simulink model "closedloop2017"  (R2017b)
settings: Solver=FixedStepAuto  StartTime=0.0  StopTime=inf  RelTol=1e-3
libraries: arduinolib x3, simulink x1
settings Model: ExtModeTrigDuration=2  Creator=colpari  LastModifiedBy=colpari
settings DataIOCC: ReturnWorkspaceOutputs=on
settings OptimizationCC: EnhancedBackFolding=on  PassReuseOutputArgsAs=Individual arguments  ZeroExternalMemoryAtStartup=off  ZeroInternalMemoryAtStartup=off  MaxStackSize=64  OptimizeBlockOrder=speed  DifferentSizesBufferReuse=on
settings DebuggingCC: ParameterTunabilityLossMsg=error
settings HardwareCC: ProdBitPerInt=16  ProdBitPerPointer=16  ProdBitPerSizeT=16  ProdBitPerPtrDiffT=16  ProdLargestAtomicFloat=None  ProdWordSize=8  ProdHWDeviceType=Atmel->AVR  UseEmbeddedCoderFeatures=off
settings SFSimCC: SimUseLocalCustomCode=on  MATLABDynamicMemAlloc=off
settings RTWCC: SystemTargetFile=ert.tlc  HardwareBoard=Arduino Uno  TLCOptions=-aInlineSetEventsForThisBaseRateFcn=TLC_FALSE -aSuppressMultiTaskScheduler=TLC_FALSE -aRateBasedStepFcn=1  TemplateMakefile=ert_default_tmf  RTWUseLocalCustomCode=on  Toolchain=Arduino AVR
settings CodeAppCC: ForceParamTrailComments=on  IgnoreCustomStorageClasses=off  OperatorAnnotations=on  SimulinkDataObjDesc=on  SFDataObjDesc=on  InsertBlockDesc=on
settings ERTTargetCC: SupportContinuousTime=on  SupportNonInlinedSFcns=on  SupportVariableSizeSignals=on  ExtModeStaticAllocSize=250

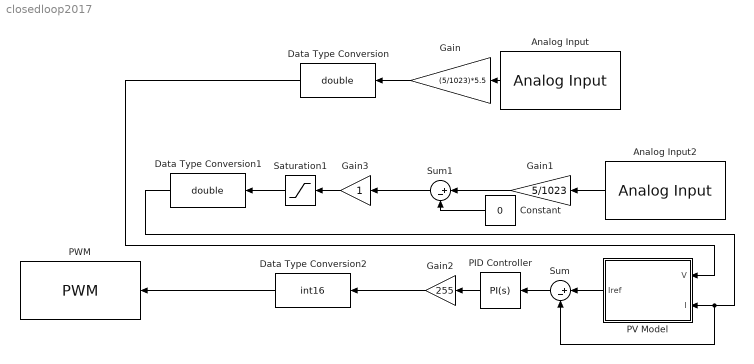
== system closedloop2017 ==
  Analog Input : arduinolib/Analog Input  pinNumber=4  ReadResultsOnly=off  ConversionTriggerSource=Software  ExternalTriggerType=uint32( 0 )  OutputDataType=uint16  EnableConversionCompleteNotify=off  EnableOuputStatus=off  SampleTime=-1  blockPlatform=arduino
  Analog Input2 : arduinolib/Analog Input  pinNumber=5  ReadResultsOnly=off  ConversionTriggerSource=Software  ExternalTriggerType=uint32( 0 )  OutputDataType=uint16  EnableConversionCompleteNotify=off  EnableOuputStatus=off  SampleTime=-1  blockPlatform=arduino
  Constant : Constant  Value=0
  Data Type Conversion : DataTypeConversion  OutDataTypeStr=double
  Data Type Conversion1 : DataTypeConversion  OutDataTypeStr=double
  Data Type Conversion2 : DataTypeConversion  OutDataTypeStr=int16
  Gain : Gain  Gain=(5/1023)*5.5
  Gain1 : Gain  Gain=5/1023
  Gain2 : Gain  Gain=255
  Gain3 : Gain
  PID Controller : simulink/Continuous/PID Controller  Controller=PI  Form=Parallel  TimeDomain=Continuous-time  SampleTime=-1  IntegratorMethod=Forward Euler  FilterMethod=Forward Euler  ControllerParametersSource=internal  P=7  I=0.003  D=0  UseFilter=on  N=100  TunerSelectOption=Transfer Function Based (PID Tuner App)  InitialConditionSource=internal  InitialConditionForIntegrator=0  InitialConditionForFilter=0  DifferentiatorICPrevScaledInput=0  ExternalReset=none  TrackingMode=off  Kt=1  LimitOutput=on  UpperSaturationLimit=1  LowerSaturationLimit=0  LinearizeAsGain=on  AntiWindupMode=none  Kb=1  POutMin=[]  POutMax=[]  IOutMin=[]  IOutMax=[]  DOutMin=[]  DOutMax=[]  NOutMin=[]  NOutMax=[]  SumOutMin=[]  SumOutMax=[]  SaturationOutMin=[]  SaturationOutMax=[]  PParamMin=[]  PParamMax=[]  IParamMin=[]  IParamMax=[]  DParamMin=[]  DParamMax=[]  NParamMin=[]  NParamMax=[]  KbParamMin=[]  KbParamMax=[]  KtParamMin=[]  KtParamMax=[]  KbOutMin=[]  KbOutMax=[]  KtOutMin=[]  KtOutMax=[]  IntegratorOutMin=[]  IntegratorOutMax=[]  FilterOutMin=[]  FilterOutMax=[]  SumI1OutMin=[]  SumI1OutMax=[]  SumI2OutMin=[]  SumI2OutMax=[]  SumI3OutMin=[]  SumI3OutMax=[]  SumDOutMin=[]  SumDOutMax=[]  DifferentiatorOutMin=[]  DifferentiatorOutMax=[]  FilterDiffOutCoefMin=[]  FilterDiffOutCoefMax=[]  ReciprocalOutMin=[]  ReciprocalOutMax=[]  SumDenOutMin=[]  SumDenOutMax=[]  SumNumOutMin=[]  SumNumOutMax=[]  DivideOutMin=[]  DivideOutMax=[]  IntegratorContinuousStateAttributes=''  IntegratorStateMustResolveToSignalObject=off  IntegratorRTWStateStorageClass=Auto  FilterContinuousStateAttributes=''  FilterStateMustResolveToSignalObject=off  FilterRTWStateStorageClass=Auto  InitialConditionSetting=State (most efficient)
  PV Model : Subsystem
  PWM : arduinolib/PWM  pinNumber=11  frequencyType=Specify  desiredFrequency=3921.16  achievableFrequency=3921.16
  Saturation1 : Saturate  LowerLimit=0
  Sum : Sum  Inputs=|+-
  Sum1 : Sum  Inputs=|+-
  wires:
  Analog Input/1 -> Gain/1
  Analog Input2/1 -> Gain1/1
  Gain/1 -> Data Type Conversion/1
  Saturation1/1 -> Data Type Conversion1/1
  Data Type Conversion2/1 -> PWM/1
  Gain2/1 -> Data Type Conversion2/1
  PID Controller/1 -> Gain2/1
  Data Type Conversion/1 -> PV Model/1(V)
  Data Type Conversion1/1 -> Sum/2, PV Model/2(I)
  PV Model/1(Iref) -> Sum/1
  Sum/1 -> PID Controller/1
  Gain3/1 -> Saturation1/1
  Constant/1 -> Sum1/2
  Gain1/1 -> Sum1/1
  Sum1/1 -> Gain3/1

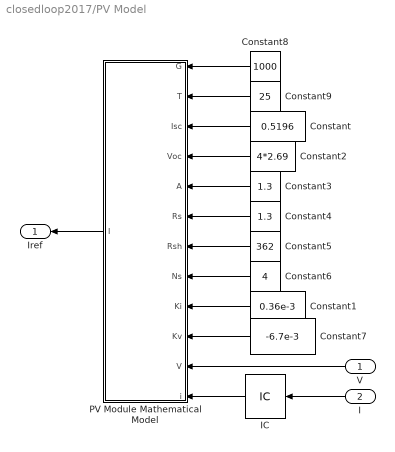
== system closedloop2017/PV Model ==
  V : Inport
  I : Inport  Port=2
  Constant : Constant  Value=0.5196
  Constant1 : Constant  Value=0.36e-3
  Constant2 : Constant  Value=4*2.69
  Constant3 : Constant  Value=1.3
  Constant4 : Constant  Value=1.3
  Constant5 : Constant  Value=362
  Constant6 : Constant  Value=4
  Constant7 : Constant  Value=-6.7e-3
  Constant8 : Constant  Value=1000
  Constant9 : Constant  Value=25
  IC : InitialCondition  Value=0
  PV Module Mathematical Model : MATLAB Function  TreatAsAtomicUnit=on
  Iref : Outport
  wires:
  Constant/1 -> PV Module Mathematical Model/3(Isc)
  Constant7/1 -> PV Module Mathematical Model/10(Kv)
  V/1 -> PV Module Mathematical Model/11(V)
  Constant5/1 -> PV Module Mathematical Model/7(Rsh)
  Constant6/1 -> PV Module Mathematical Model/8(Ns)
  Constant1/1 -> PV Module Mathematical Model/9(Ki)
  Constant8/1 -> PV Module Mathematical Model/1(G)
  Constant4/1 -> PV Module Mathematical Model/6(Rs)
  Constant2/1 -> PV Module Mathematical Model/4(Voc)
  IC/1 -> PV Module Mathematical Model/12(i)
  Constant9/1 -> PV Module Mathematical Model/2(T)
  Constant3/1 -> PV Module Mathematical Model/5(A)
  PV Module Mathematical Model/1(I) -> Iref/1
  I/1 -> IC/1

== matlab function closedloop2017/PV Model/PV Module Mathematical Model ==
  data: G input; T input; Isc input; Voc input; A input; Rs input; Rsh input; Ns input; Ki input; Kv input; V input; i input; I output
function I = fcn(G,T,Isc,Voc,A,Rs,Rsh,Ns,Ki,Kv,V,i)
    
    q = 1.6e-19;                          % Electron charge
    k = 1.38e-23;                         % Boltzmann constant
    Tcell = 273+T;                        % Cell temperature in Kelvin
    vt=(A*k*Tcell*Ns)/q;                  % Thermal voltage Equation(5)
        
    Isc_T = Isc+((Isc*(Ki/100))*(T-25));  % Isc temperature coef Equation(6)
    Voc_T = Voc+((Voc*(Kv/100))*(T-25));  % Voc temperature coef Equation(7)
    Is = Isc_T/(exp(Voc_T/vt)-1);         % Reverse saturation current Equation(8)
    Iph = Isc_T*(G/1000);                 % Photon current Equation(9)
    
    % Single diode model output current Equation(4)
    I = Iph-(Is*(exp((V+(i*Rs))/vt)-1))-((V+(i*Rs))/Rsh);
end
